simulink model "Exercicio_4_2_Vinicius"  (R2015a)
settings: Solver=ode45  StartTime=0.0  StopTime=3  FixedStep=Ts  RelTol=1e-3
undefined symbols (not defined in the file): AA, BB, DD, H, KE, KF, KR, Ts
libraries: cstblocks x1
settings Model: Creator=vinic  LastModifiedBy=vinic

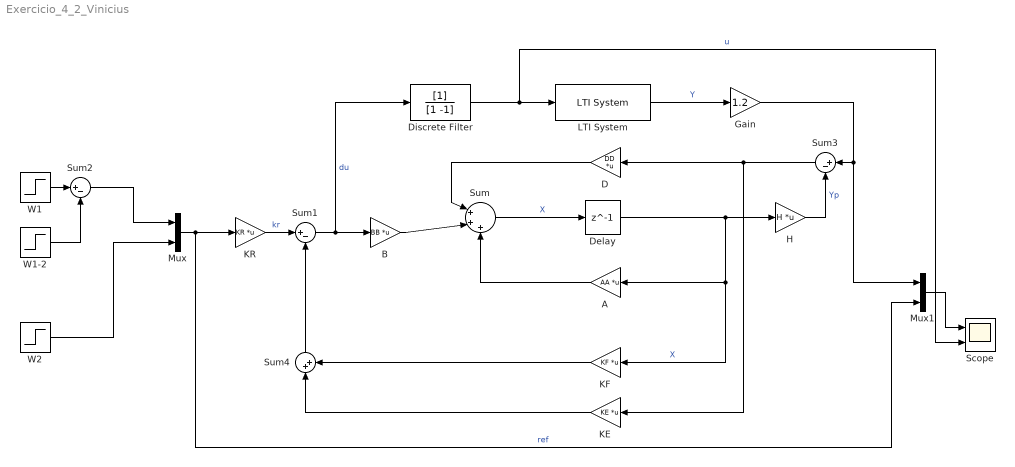
== system Exercicio_4_2_Vinicius ==
  A : Gain  Gain=AA  Multiplication=Matrix(K*u)
  B : Gain  Gain=BB  Multiplication=Matrix(K*u)
  D : Gain  Gain=DD  Multiplication=Matrix(K*u)
  Delay : Delay  DelayLength=1  SampleTime=Ts
  Discrete Filter : DiscreteFilter  Denominator=[1 -1]  SampleTime=Ts
  Gain : Gain  Gain=1.2
  H : Gain  Gain=H  Multiplication=Matrix(K*u)
  KE : Gain  Gain=KE  Multiplication=Matrix(K*u)
  KF : Gain  Gain=KF  Multiplication=Matrix(K*u)
  KR : Gain  Gain=KR  Multiplication=Matrix(K*u)
  LTI System : cstblocks/LTI System  sys=Cd  IC=[]
  Mux : Mux  Inputs=2
  Mux1 : Mux  Inputs=2
  Scope : Scope  NumInputPorts=2
      settings: YMin=0~-5  YMax=0.6~5  SaveName=simul
  Sum : Sum  Inputs=|+++
  Sum1 : Sum  Inputs=|+-
  Sum2 : Sum  Inputs=|+-
  Sum3 : Sum  Inputs=|+-
  Sum4 : Sum  Inputs=|++
  W1 : Step  Time=0  After=0.5  SampleTime=Ts
  W1-2 : Step  Time=1.5  After=0.1  SampleTime=Ts
  W2 : Step  Time=0  After=0.3  SampleTime=Ts
  wires:
  Sum/1 -> Delay/1  "X"
  Delay/1 -> KF/1, A/1, H/1  "X"
  LTI System/1 -> Gain/1  "Y"
  A/1 -> Sum/3
  B/1 -> Sum/2
  D/1 -> Sum/1
  Sum3/1 -> KE/1, D/1
  Sum1/1 -> Discrete Filter/1, B/1  "du"
  H/1 -> Sum3/2  "Yp"
  Discrete Filter/1 -> Scope/2, LTI System/1  "u"
  KE/1 -> Sum4/1
  KF/1 -> Sum4/2
  Sum4/1 -> Sum1/2
  Mux/1 -> Mux1/2, KR/1  "ref"
  KR/1 -> Sum1/1  "kr"
  W2/1 -> Mux/2
  W1/1 -> Sum2/1
  Sum2/1 -> Mux/1
  W1-2/1 -> Sum2/2
  Mux1/1 -> Scope/1
  Gain/1 -> Mux1/1, Sum3/1
